simulink model "Model"  (R2020b)
settings: Solver=VariableStepAuto  StartTime=0.0  StopTime=10.0  RelTol=1e-3
values from neighbouring files (symbols this model uses):
  R_r = 11.78    [parameters.m]
  R_s = 13.2    [parameters.m]
settings Model: Creator=Basilisk  LastModifiedBy=Basilisk

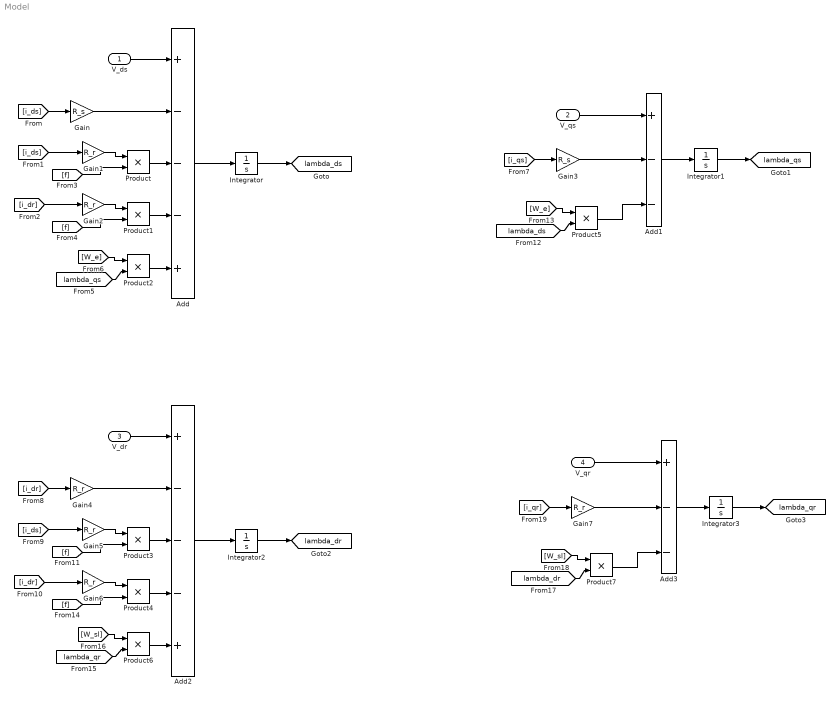
== system Model ==
  V_ds : Inport
  V_qs : Inport  Port=2
  V_dr : Inport  Port=3
  V_qr : Inport  Port=4
  Add : Sum  Inputs=+---+
  Add1 : Sum  Inputs=+--
  Add2 : Sum  Inputs=+---+
  Add3 : Sum  Inputs=+--
  Gain : Gain  Gain=R_s
  Gain{1..2,4..7} (6 alike) : Gain  Gain=R_r
  Gain3 : Gain  Gain=R_s
  Integrator{,1..3} (4 alike) : Integrator
  Product{,1..7} (8 alike) : Product
  tag scope: lambda_dr=global, lambda_ds=global, lambda_qr=global, lambda_qs=global
  wires:
  [i_ds] -> Gain/1
  Gain/1 -> Add/2
  V_ds/1 -> Add/1
  [i_ds] -> Gain1/1
  Product/1 -> Add/3
  Gain1/1 -> Product/1
  [f] -> Product/2
  Product1/1 -> Add/4
  Gain2/1 -> Product1/1
  [i_dr] -> Gain2/1
  [f] -> Product1/2
  Product2/1 -> Add/5
  [W_e] -> Product2/1
  [lambda_qs] -> Product2/2
  Add/1 -> Integrator/1
  Integrator/1 -> [lambda_ds]
  Integrator1/1 -> [lambda_qs]
  [lambda_ds] -> Product5/2
  V_qs/1 -> Add1/1
  Product5/1 -> Add1/3
  Gain3/1 -> Add1/2
  Add1/1 -> Integrator1/1
  [W_e] -> Product5/1
  [i_qs] -> Gain3/1
  Integrator2/1 -> [lambda_dr]
  [f] -> Product3/2
  Product3/1 -> Add2/3
  [lambda_qr] -> Product6/2
  V_dr/1 -> Add2/1
  Product6/1 -> Add2/5
  Product4/1 -> Add2/4
  Gain6/1 -> Product4/1
  Gain4/1 -> Add2/2
  Add2/1 -> Integrator2/1
  [W_sl] -> Product6/1
  [f] -> Product4/2
  Gain5/1 -> Product3/1
  [i_ds] -> Gain5/1
  [i_dr] -> Gain6/1
  [i_dr] -> Gain4/1
  [W_sl] -> Product7/1
  [i_qr] -> Gain7/1
  Gain7/1 -> Add3/2
  V_qr/1 -> Add3/1
  Integrator3/1 -> [lambda_qr]
  Add3/1 -> Integrator3/1
  [lambda_dr] -> Product7/2
  Product7/1 -> Add3/3
